simulink model "Quanser_Qube_Plant_Model_Check"  (R2019a)
settings: Solver=VariableStepAuto  StartTime=0.0  StopTime=10.0  RelTol=1e-3
libraries: cstblocks x1
settings Model: Creator=emma  LastModifiedBy=emma

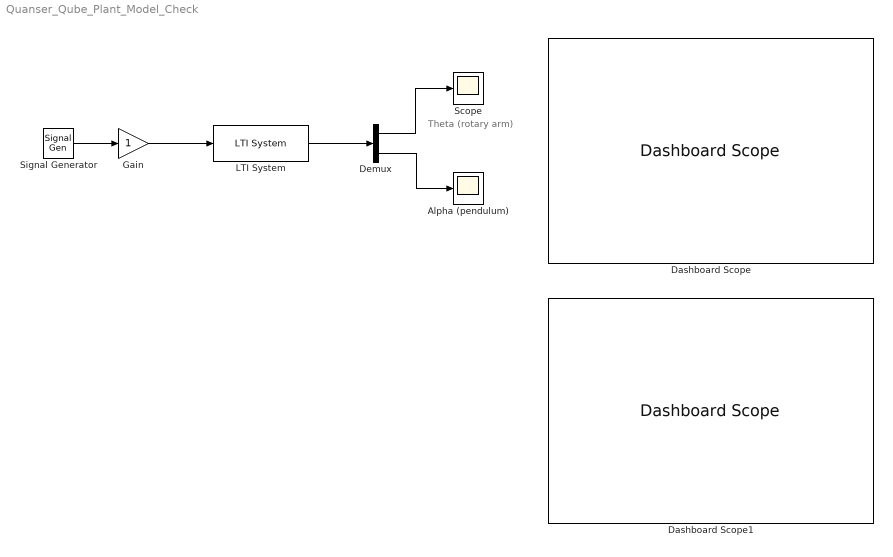
== system Quanser_Qube_Plant_Model_Check ==
  note: Theta (rotary arm)
  Alpha (pendulum) : Scope
  Dashboard Scope : DashboardScope
  Dashboard Scope1 : DashboardScope
  Demux : Demux  Outputs=2
  Gain : Gain
  LTI System : cstblocks/LTI System  sys=Galt  IC=[]
  Scope : Scope
  Signal Generator : SignalGenerator  Frequency=6.28  Units=rad/sec
  wires:
  Signal Generator/1 -> Gain/1
  Gain/1 -> LTI System/1
  LTI System/1 -> Demux/1
  Demux/1 -> Scope/1
  Demux/2 -> Alpha (pendulum)/1
